simulink model "quadrotor_stage2"  (R2026a)
settings: Solver=ode45  StopTime=15  MaxStep=0.005  RelTol=1e-6
settings Model: Creator=ASUS  LastModifiedBy=ASUS

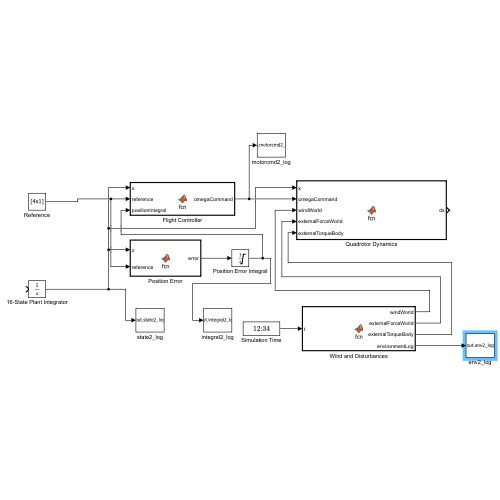
[thumbnail: Simulink's stored preview of the top-level diagram]
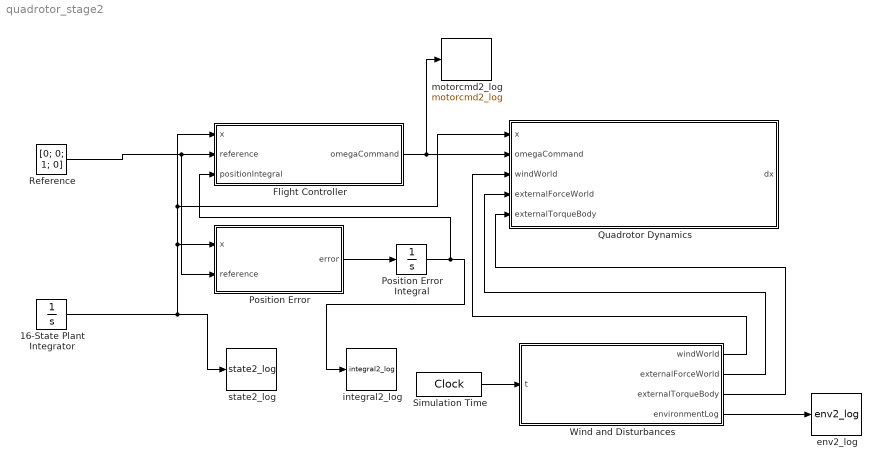
== system quadrotor_stage2 ==
  16-State Plant Integrator : Integrator  InitialCondition=[zeros(12,1); sqrt(1.20*9.81/(4*1.8e-5))*ones(4,1)]
  Flight Controller : MATLAB Function  TreatAsAtomicUnit=on
  Position Error : MATLAB Function  TreatAsAtomicUnit=on
  Position Error Integral : Integrator  InitialCondition=zeros(3,1)  LimitOutput=on  UpperSaturationLimit=[4;4;1.5]  LowerSaturationLimit=[-4;-4;-1.5]
  Quadrotor Dynamics : MATLAB Function  TreatAsAtomicUnit=on
  Reference : Constant  Value=[0; 0; 1; 0]
  Simulation Time : DigitalClock
  Wind and Disturbances : MATLAB Function  TreatAsAtomicUnit=on
  env2_log : ToWorkspace  VariableName=env2_log  SaveFormat=Timeseries  SampleTime=-1
      settings: Save2DSignal=2-D array (concatenate along first dimension)
  integral2_log : ToWorkspace  VariableName=integral2_log  SaveFormat=Timeseries  SampleTime=-1
      settings: Save2DSignal=2-D array (concatenate along first dimension)
  motorcmd2_log : ToWorkspace  VariableName=motorcmd2_log  SaveFormat=Timeseries  SampleTime=-1
      settings: Save2DSignal=2-D array (concatenate along first dimension)
  state2_log : ToWorkspace  VariableName=state2_log  SaveFormat=Timeseries  SampleTime=-1
      settings: Save2DSignal=2-D array (concatenate along first dimension)
  wires:
  Reference/1 -> Position Error/2(reference), Flight Controller/2(reference)
  Flight Controller/1(omegaCommand) -> motorcmd2_log/1, Quadrotor Dynamics/2(omegaCommand)
  16-State Plant Integrator/1 -> state2_log/1, Position Error/1(x), Flight Controller/1(x), Quadrotor Dynamics/1(x)
  Position Error/1(error) -> Position Error Integral/1
  Position Error Integral/1 -> integral2_log/1, Flight Controller/3(positionIntegral)
  Simulation Time/1 -> Wind and Disturbances/1(t)
  Wind and Disturbances/1(windWorld) -> Quadrotor Dynamics/3(windWorld)
  Wind and Disturbances/2(externalForceWorld) -> Quadrotor Dynamics/4(externalForceWorld)
  Wind and Disturbances/3(externalTorqueBody) -> Quadrotor Dynamics/5(externalTorqueBody)
  Wind and Disturbances/4(environmentLog) -> env2_log/1

== matlab function quadrotor_stage2/Quadrotor Dynamics ==
  data: x input; dx output; omegaCommand input; windWorld input; externalForceWorld input; externalTorqueBody input
function dx = fcn(x, omegaCommand, windWorld, ...
    externalForceWorld, externalTorqueBody)
%#codegen
dx = quadDynamicsStage2(x, omegaCommand, windWorld, ...
    externalForceWorld, externalTorqueBody);
end

== matlab function quadrotor_stage2/Flight Controller ==
  data: x input; omegaCommand output; reference input; positionIntegral input
function omegaCommand = fcn(x, reference, positionIntegral)
%#codegen
omegaCommand = flightControllerStage2(x, reference, positionIntegral);
end

== matlab function quadrotor_stage2/Position Error ==
  data: x input; error output; reference input
function error = fcn(x, reference)
%#codegen
error = reference(1:3) - x(1:3);
end

== matlab function quadrotor_stage2/Wind and Disturbances ==
  data: t input; windWorld output; externalForceWorld output; externalTorqueBody output; environmentLog output
function [windWorld, externalForceWorld, ...
    externalTorqueBody, environmentLog] = fcn(t)
%#codegen
[windWorld, externalForceWorld, externalTorqueBody, environmentLog] = ...
    environmentStage2(t);
end
